simulink model "two_link"  (Simulink 8.7)
settings: Solver=VariableStepAuto  StartTime=0.0  StopTime=20  RelTol=1e-3
undefined symbols (not defined in the file or in its folder): call_two_link, external_cal, external_cal_resi_dera, P_cal, two_link_gravity_position_control
libraries: simulink x2
settings Model: Creator=Godric  LastModifiedBy=Godric
settings DataIOCC: LimitDataPoints=off  SaveFormat=Dataset
settings DebuggingCC: UnderspecifiedInitializationDetection=Simplified  MergeDetectMultiDrivingBlocksExec=error
settings HardwareCC: ProdBitPerPointer=64  ProdLargestAtomicFloat=Float  ProdIntDivRoundTo=Zero  ProdEndianess=LittleEndian  ProdWordSize=64  ProdHWDeviceType=Intel->x86-64 (Windows64)
settings ModelReferenceCC: PropagateSignalLabelsOutOfModel=on
settings ConfigComp: CovModelRefEnable=off

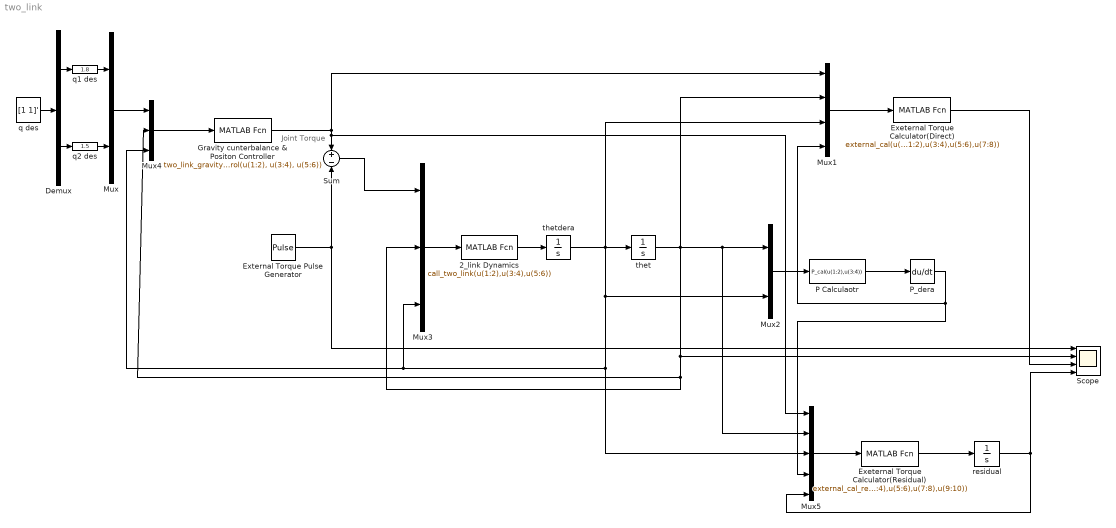
== system two_link ==
  note: Joint Torque
  2_link Dynamics : MATLABFcn  MATLABFcn=call_two_link(u(1:2),u(3:4),u(5:6))  OutputDimensions=[2,1]  Output1D=off
  Demux : Demux  Outputs=2
  Exeternal Torque Calculator(Direct) : MATLABFcn  MATLABFcn=external_cal(u(1:2),u(3:4),u(5:6),u(7:8))  OutputDimensions=[2,1]  Output1D=off
  Exeternal Torque Calculator(Residual) : MATLABFcn  MATLABFcn=external_cal_resi_dera(u(1:2),u(3:4),u(5:6),u(7:8),u(9:10))  OutputDimensions=[2,1]  Output1D=off
  External Torque Pulse Generator : DiscretePulseGenerator  PulseType=Time based  Amplitude=[2.8 10]'  Period=20  PulseWidth=2  PhaseDelay=3
  Gravity cunterbalance & Positon Controller : MATLABFcn  MATLABFcn=two_link_gravity_position_control(u(1:2), u(3:4), u(5:6))  OutputDimensions=[2,1]  Output1D=off
  Mux : Mux  Inputs=2
  Mux1 : Mux
  Mux2 : Mux  Inputs=2
  Mux3 : Mux  Inputs=3
  Mux4 : Mux  Inputs=3
  Mux5 : Mux  Inputs=5
  P Calculaotr : MATLABFcn  MATLABFcn=P_cal(u(1:2),u(3:4))  OutputDimensions=[2,1]  Output1D=off
  P_dera : Derivative
  Scope : Scope  NumInputPorts=4
  Sum : Sum  Inputs=+-
  q des : Constant  Value=[1 1]'
  q1 des : simulink/Math Operations/Slider Gain  low=-2  gain=1.8  high=2
  q2 des : simulink/Math Operations/Slider Gain  low=-2  gain=1.5  high=2
  residual : Integrator
  thet : Integrator
  thetdera : Integrator
  wires:
  Mux3/1 -> 2_link Dynamics/1
  Sum/1 -> Mux3/1
  2_link Dynamics/1 -> thetdera/1
  thet/1 -> Mux5/2, Mux2/1, Scope/2, Mux4/2, Mux3/2, Mux1/2
  Mux1/1 -> Exeternal Torque Calculator(Direct)/1
  thetdera/1 -> Mux1/3, Mux2/2, Mux5/3, Mux4/3, Mux3/3, thet/1
  External Torque Pulse Generator/1 -> Sum/2, Scope/1
  Mux2/1 -> P Calculaotr/1
  P Calculaotr/1 -> P_dera/1
  P_dera/1 -> Mux5/4, Mux1/4
  Demux/1 -> q1 des/1
  Demux/2 -> q2 des/1
  q2 des/1 -> Mux/2
  q1 des/1 -> Mux/1
  q des/1 -> Demux/1
  Mux/1 -> Mux4/1
  Mux4/1 -> Gravity cunterbalance & Positon Controller/1
  Gravity cunterbalance & Positon Controller/1 -> Mux5/1, Sum/1, Mux1/1
  Exeternal Torque Calculator(Direct)/1 -> Scope/3
  Mux5/1 -> Exeternal Torque Calculator(Residual)/1
  Exeternal Torque Calculator(Residual)/1 -> residual/1
  residual/1 -> Scope/4, Mux5/5
